simulink model "untitled2"  (R2019a)
settings: Solver=VariableStepAuto  StartTime=0.0  StopTime=10.0  RelTol=1e-3
undefined symbols (not defined in the file or in its folder): T
libraries: simulink_extras x1
settings Model: Creator=Sagar  LastModifiedBy=Sagar

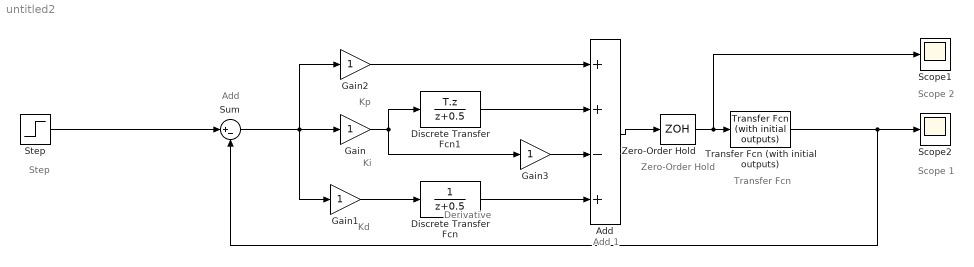
== system untitled2 ==
  note: Zero-Order Hold
  note: Step
  note: Kd
  note: Add 1
  note: Scope 1
  note: Derivative
  note: Add
  note: Ki
  note: Transfer Fcn
  note: Kp
  note: Scope 2
  Add : Sum  Inputs=++-+
  Discrete Transfer Fcn : DiscreteTransferFcn
  Discrete Transfer Fcn1 : DiscreteTransferFcn  Numerator=T.z
  Gain{,1..3} (4 alike) : Gain
  Scope1 : Scope
  Scope2 : Scope
  Step : Step  SampleTime=0
  Sum : Sum  Inputs=|+-
  Transfer Fcn (with initial outputs) : simulink_extras/Additional Linear/Transfer Fcn (with initial outputs)  N=[1]  D="[1  20 20]"  Y0=.5  U0=0
  Zero-Order Hold : ZeroOrderHold  SampleTime=-1
  wires:
  Sum/1 -> Gain1/1, Gain2/1, Gain/1
  Discrete Transfer Fcn/1 -> Add/4
  Gain1/1 -> Discrete Transfer Fcn/1
  Transfer Fcn (with initial outputs)/1 -> Scope2/1, Sum/2
  Gain2/1 -> Add/1
  Add/1 -> Zero-Order Hold/1
  Step/1 -> Sum/1
  Gain/1 -> Gain3/1, Discrete Transfer Fcn1/1
  Zero-Order Hold/1 -> Scope1/1, Transfer Fcn (with initial outputs)/1
  Discrete Transfer Fcn1/1 -> Add/2
  Gain3/1 -> Add/3
